simulink model "Project2Question2_AkankshaMurali"  (R2023b)
settings: Solver=VariableStepAuto  StartTime=0.0  StopTime=10.0  RelTol=1e-3
settings Model: Creator=angel  LastModifiedBy=akank
settings RTWCC: GPUComputeCapability=5.0

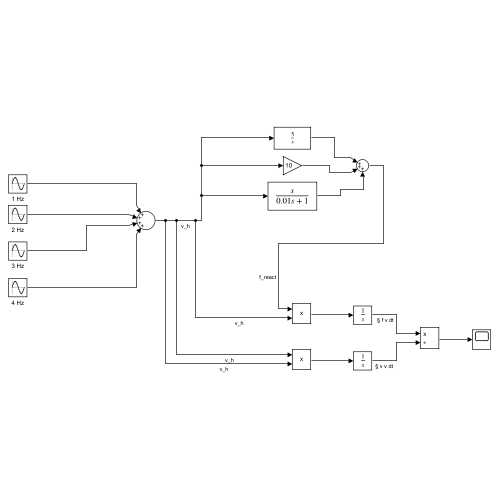
[thumbnail: Simulink's stored preview of the top-level diagram]
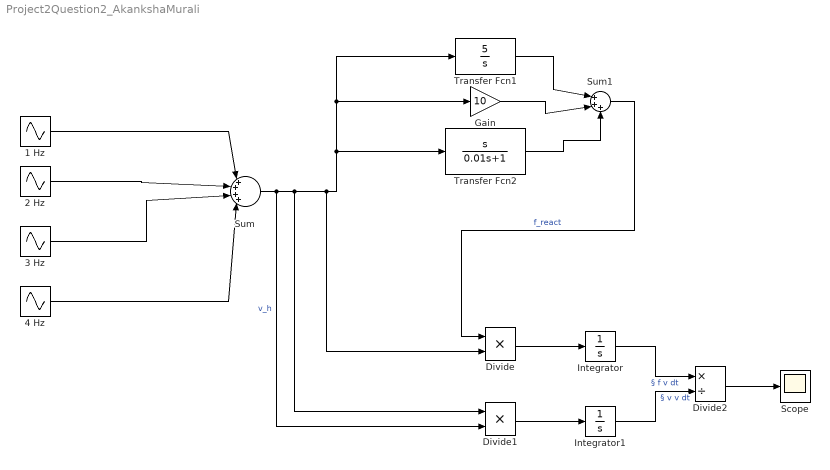
== system Project2Question2_AkankshaMurali ==
  1 Hz : Sin  Frequency=1 * 2* pi  SampleTime=0
  2 Hz : Sin  Frequency=2 * 2 * pi  SampleTime=0
  3 Hz : Sin  Frequency=3 * 2 * pi  SampleTime=0
  4 Hz : Sin  Frequency=4 * 2 * pi  SampleTime=0
  Divide : Product  Inputs=**
  Divide1 : Product  Inputs=**
  Divide2 : Product  Inputs=*/
  Gain : Gain  Gain=10
  Integrator : Integrator
  Integrator1 : Integrator
  Scope : Scope
  Sum : Sum  Inputs=|++++|
  Sum1 : Sum  Inputs=|+++
  Transfer Fcn1 : TransferFcn  Numerator=[5]  Denominator=[1 0]
  Transfer Fcn2 : TransferFcn  Numerator=[1 0]  Denominator=[0.01 1]
  wires:
  1 Hz/1 -> Sum/1
  2 Hz/1 -> Sum/2
  3 Hz/1 -> Sum/3
  4 Hz/1 -> Sum/4
  Sum/1 -> Divide1/2, Divide1/1, Divide/2, Transfer Fcn2/1, Gain/1, Transfer Fcn1/1  "v_h"
  Sum1/1 -> Divide/1  "f_react"
  Divide/1 -> Integrator/1
  Integrator/1 -> Divide2/1  "§ f v dt"
  Divide1/1 -> Integrator1/1
  Integrator1/1 -> Divide2/2  "§ v v dt"
  Divide2/1 -> Scope/1
  Transfer Fcn2/1 -> Sum1/3
  Gain/1 -> Sum1/2
  Transfer Fcn1/1 -> Sum1/1
